simulink library "xbsDSP48_r3"  (Simulink 5.0)
libraries: xbsIndex_r3 x429, xbsDSP48_r3 x2
(part 2 of 8)

== system xbsDSP48_r3/DSP48_Adder ==
  note: A and C Type Casting : No Cost in Hardware
  note: Carry in Select Mux : From Fabric or no Carry in
  note: Output P Type Casting to  User Defined
      | Data Type
  In1 : Inport
  In3 : Inport  Port=2
  In6 : Inport  Port=3
  A : xbsIndex_r3/Slice  mode=Upper Bit Location + Width  nbits=18  bit1=0  base1=MSB of Input  bit0=0  base0=LSB of Input  boolean_output=off  explicit_period=off  period=1  dbl_ovrd=off
  AlignA : S-Function  AncestorBlock=xbsIndex_r3/Convert  FunctionName=xlconvert  Parameters=sfcn_mwsv__  mask(Xilinx Converter Block){arith_type=Signed  (2's comp), n_bits=15, bin_pt=0, quantization=Truncate, overflow=Wrap, latency=0, explicit_period=off, period=1, dbl_ovrd=off, show_param=off, inserted_by_tool=off, xl_area=[0, 0, 0, 0, 0, 0, 0], xl_use_area=off}
      mask prompts: arith_type "Output Type"; n_bits "Number of Bits"; bin_pt "Binary Point"; quantization "Quantization Behavior"; overflow "Overflow Behavior"; explicit_period "Use Explicit Sample Period"; period "Sample Period"; dbl_ovrd "Override with Doubles"; show_param "---------------------- Show Implementation Parameters -----------------------------------------------------------------------------------"; inserted_by_tool "Hidden Parameter:  inserted_by_tool"; xl_area "FPGA Area [Slices, FFs, BRAMs, LUTs, IOBs, Emb. Mults, TBUFs]"; xl_use_area "Use Area Above For Estimation"
      mask help:
      | Type conversion block. The input is presented at the output after quantization and overflow effects.
      |
      | Hardware notes: Additional hardware is used when rounding or saturation is selected and output width is less than the input width.
      mask init:
      | [designRoot, family, part, speed, package, simulinkPeriod, sysclkPeriod, dbl_ovrd, trimVbit] = xlSysgenSettings(gcb,1,1);
      | if (arith_type==1)
      |   bool = 1;
      | else
      |   bool = 0;
      |   arith_type = arith_type-1;
      | end
      | zstr=''; zpstr='';
      | if latency > 0
      |   zstr = 'z';
      |   zpstr = sprintf('-%d', latency);
      | end
      | [bg,fg] = xlcmap('XBlock',dbl_ovrd);
      | if (inserted_by_tool)
      |   bg = [1.00 0.50 0.25];
      | end
      | iPos = get_param(gcb,'Position');
      | iWidth=iPos(3)-iPos(1); iHeight=iPos(4)-iPos(2);
      | iCx=iWidth/2;
      | iCy=iHeight/2;
      | [logoX, logoY] = xlogo(iPos);
      | zstrx = 0.45*iWidth-11; if (zstrx<3) zstrx=3; end
      | zstry = 0.36*iHeight-7; if (zstry<3) zstry=3; end
      | 
      | 
      | % one time added for param list
      | dblOvrd = dbl_ovrd;
      | precision0 = 2;
      | z0 = [n_bits bin_pt arith_type quantization overflow];
      | explicitClk = explicit_period;
      | 
      | 
      | % just pass everything to s-function
      | sfcn_mwsv__ = get_param(gcb, 'MaskWSVariables');
      mask Help: web(xlhtmldoclink('Convert'));
      mask StyleString: popup(Boolean|Unsigned|Signed  (2's comp)),edit,edit,popup(Truncate|Round  (unbiased: +/- Inf)|Round  (unbiased: Even Values)),popup(Wrap|Saturate|Error),edit,checkbox,edit,checkbox,checkbox,checkbox,edit,checkbox
      mask Display:
      | patch([0 iWidth iWidth 0],[0 0 iHeight iHeight] , bg);
      | patch(logoX,logoY , fg);
      | text(zstrx,zstry,zstr);
      | text(zstrx+5,zstry+5,zpstr);
      | port_label('output',1,'cast');
      | plot([0 0 iWidth iWidth 0], [0 iHeight iHeight 0 0]);
  AlignC : xbsIndex_r3/Convert  arith_type="Signed  (2's comp)"  n_bits=12  bin_pt=0  quantization=Truncate  overflow=Wrap  latency=0  explicit_period=off  period=1  dbl_ovrd=off  show_param=off  inserted_by_tool=off  pipeline=off
      settings: xl_area=[0, 0, 0, 0, 0, 0, 0]
  AlignP : xbsIndex_r3/Reinterpret  force_arith_type=off  arith_type=Unsigned  force_bin_pt=on  bin_pt=0  force_valid=on
  B : xbsIndex_r3/Slice  mode=Lower Bit Location + Width  nbits=18  bit1=0  base1=MSB of Input  bit0=0  base0=LSB of Input  boolean_output=off  explicit_period=off  period=1  dbl_ovrd=off
  ConvertP : xbsIndex_r3/Convert  arith_type="Signed  (2's comp)"  n_bits=48  bin_pt=0  quantization=Truncate  overflow=Wrap  latency=0  explicit_period=off  period=1  dbl_ovrd=off  show_param=off  inserted_by_tool=off  pipeline=off
      settings: xl_area=[0, 0, 0, 0, 0, 0, 0]
  DSP48 : S-Function  FunctionName=xldsp48  Parameters=sfcn_mwsv__  mask(Xilinx DSP48){pipeline_a=1, use_b=Direct from B Port, pipeline_b=1, pipeline_bcin=0, pipeline_c=on, pipeline_p=on, pipeline_mult=on, pipeline_opmode=on, pipeline_sub=on, pipeline_carryin=on, pipeline_carryinsel=on, use_op=off, use_creg=on, use_pcin=off, use_pcout=off, use_bcout=off, access_rst=off, rst_all=off, rst_a=off, rst_b=off, rst_bcin=off, rst_c=off, rst_p=off, rst_mult=off, rst_carry_in=off, rst_ctrl=off, access_en=off, en_all=off, en_a=off, en_b=off, en_bcin=off, en_c=off, en_p=off, en_mult=off, en_carry_in=off, en_ctrl=off, explicit_period=off, period=1, dbl_ovrd=off, xl_area=[0, 0, 0, 0, 0, 0, 0], xl_use_area=on}
      mask prompts: pipeline_a "Pipeline Input A"; use_b "B Input"; pipeline_b "Pipeline Input B"; pipeline_bcin "Pipeline Input BCIN"; pipeline_c "Pipeline Input C"; pipeline_p "Pipeline P"; pipeline_mult "Pipeline Multiplier"; pipeline_opmode "Pipeline OpMode"; pipeline_sub "Pipeline Subtract"; pipeline_carryin "Pipeline Carry In"; pipeline_carryinsel "Pipeline Carry In Sel"; use_op "Consolidate Control Port (opmode, subtract, carry_in, carry_in_sel)"; use_creg "Provide C Port"; use_pcin "Provide PCIN Port"; use_pcout "Provide PCOUT Port"; use_bcout "Provide BCOUT Port"; access_rst "---------------------- Access Reset Port Control ---------------------------------------------------------"; rst_all "Provide Global Reset Port"; rst_a "Provide Reset Port for A"; rst_b "Provide Reset Port for B"; rst_bcin "Provide Reset Port for BCIN"; rst_c "Provide Reset Port for C"; rst_p "Provide Reset Port for P"; rst_mult "Provide Reset Port for Multiplier"; rst_carry_in "Provide Reset Port for Carry In"; rst_ctrl "Provide Reset Port for Controls (Subtract, CarryInSel, OpMode)"; access_en "---------------------- Access Enable Port Controls ---------------------------------------------------------"; en_all "Provide Global Enable Port"; en_a "Provide Enable Port for A"; en_b "Provide Enable Port for B"; en_bcin "Provide Enable Port for BCIN"; en_c "Provide Enable Port for C"; en_p "Provide Enable Port for P"; en_mult "Provide Enable Port for Multiplier"; en_carry_in "Provide Enable Port for Carry In"; en_ctrl "Provide Enable Port for Controls (Subtract, CarryInSel, OpMode)"; explicit_period "Use Explicit Sample Period"; period "Sample Period  (use -1 to inherit first known input period)"; dbl_ovrd "Override with Doubles"; xl_area "FPGA Area [Slices, FFs, BRAMs, LUTs, IOBs, Emb. Mults, TBUFs]"; xl_use_area "Use Area Above For Estimation"
      mask init:
      | [designRoot, family, part, speed, package, simulinkPeriod, sysclkPeriod, dbl_ovrd, trimVbit] = xlSysgenSettings(gcb,1,0);
      | trimVbit=1;
      | [bg,fg] = xlcmap('XBlock',dbl_ovrd);
      | iPos = get_param(gcb,'Position');
      | iWidth=iPos(3)-iPos(1); iHeight=iPos(4)-iPos(2);
      | iCx=iWidth/2;
      | iCy=iHeight/2;
      | [logoX, logoY] = xlogo(iPos);
      | opt_ports = 3; % default starting port num for optional ports
      | %initialize all the strings
      | b_str = 'a'; b_num = 1;
      | c_str = 'a'; c_num = 1;
      | ce_all_str = 'a'; rst_all_str = 'a';
      | ce_a_str = 'a'; rst_a_str = 'a';
      | ce_b_str = 'a'; rst_b_str = 'a';
      | ce_c_str = 'a'; rst_c_str = 'a';
      | ce_mult_str = 'a'; rst_mult_str = 'a';
      | ce_p_str = 'a'; rst_p_str = 'a';
      | ce_ctrl_str = 'a'; rst_ctrl_str = 'a';
      | ce_carryin_str = 'a'; rst_carryin_str = 'a';
      | ce_cinsub_str = 'a'; rst_cinsub_str = 'a';
      | bcin_str = 'a'; pcin_str = 'a';
      | pcout_str = 'p'; bcout_str = 'p';
      | opstr = 'a'; sub_str = 'a'; carryin_str = 'a';
      | carryin_sel_str = 'a';
      | % initialize all the port nums
      | ce_all_num = 1; rst_all_num = 1;
      | ce_a_num = 1; rst_a_num = 1;
      | ce_b_num = 1; rst_b_num = 1;
      | ce_c_num = 1; rst_c_num = 1;
      | ce_p_num = 1; rst_p_num = 1;
      | ce_mult_num = 1; rst_mult_num = 1;
      | ce_ctrl_num = 1; rst_ctrl_num = 1;
      | ce_carryin_num = 1; rst_carryin_num = 1;
      | ce_cinsub_num = 1; rst_cinsub_num = 1;
      | bcin_num = 1; pcin_num = 1;
      | pcout_num = 1; bcout_num = 1;
      | opnum = 1; sub_num = 1;
      | carryin_num = 1; carryin_sel_num = 1;
      | %Determine output ports
      | if(use_bcout == 1)
      | 	bcout_num = 2;
      | 	bcout_str = 'bcout';
      | end
      | if(use_pcout == 1)
      | 	if(use_bcout == 1)
      | 		pcout_num = 3;
      | 	else
      | 		pcout_num = 2;
      | 	end
      | 	pcout_str = 'pcout';
      | end
      | %determine to use b or bcin
      | if(use_b == 1) % USE B
      | 	b_str = 'b';
      | 	b_num = 2;
      | end
      | if(use_b == 2) % USE BCIN - place in same location as B
      | 	bcin_num = 2;
      | 	bcin_str = 'bcin';
      | end
      | if(use_creg == 1)
      | 	c_num = 3;
      | 	opt_ports = 4;
      | 	c_str = 'c';
      | end
      | if(use_pcin == 1)
      | 	pcin_num = opt_ports;
      | 	pcin_str = 'pcin';
      | 	opt_ports = opt_ports + 1;
      | end
      | %determine to use consolidated opmode or not
      | if(use_op == 1)
      | 	opnum = opt_ports;
      | 	opt_ports = opt_ports + 1;
      | 	opstr = 'op';
      | else
      | 	opnum = opt_ports;
      | 	opstr = 'opmode';
      | 	opt_ports = opt_ports + 1;
      | 	sub_num = opt_ports;
      | 	sub_str = 'subtract';
      | 	opt_ports = opt_ports + 1;
      | 	carryin_num = opt_ports;
      | 	carryin_str = 'carry_in';
      | 	opt_ports = opt_ports + 1;
      | 	carryin_sel_num = opt_ports;
      | 	carryin_sel_str = 'carry_in_sel';
      | 	opt_ports = opt_ports + 1;
      | end
      | %determine which optional ports to display
      | if(en_all == 1)
      | 	ce_a_str = 'en';
      | 	ce_a_num = opt_ports;
      | 	opt_ports = opt_ports + 1;
      | end
      | if(pipeline_a ~= 1 & en_a == 1 & en_all == 0)
      | 	ce_a_str = 'ce_a';
      | 	ce_a_num = opt_ports;
      | 	opt_ports = opt_ports + 1;
      | end
      | if(pipeline_b ~= 1 & (en_b == 1 || en_bcin == 1) & en_all == 0)
      | 	if(en_b == 1)
      | 		ce_b_str = 'ce_b';
      | 	end
      | 	if(en_bcin == 1)
      | 		ce_b_str = 'ce_bcin';
      | 	end
      | 	ce_b_num = opt_ports;
      | 	opt_ports = opt_ports + 1;
      | end
      | if(pipeline_c == 1 & en_c == 1 & en_all == 0)
      | 	ce_c_num = opt_ports;
      | 	ce_c_str = 'ce_c';
      | 	opt_ports = opt_ports + 1;
      | end
      | if(pipeline_mult == 1 & en_mult == 1 & en_all == 0)
      | 	ce_mult_num = opt_ports;
      | 	ce_mult_str = 'ce_m';
      | 	opt_ports = opt_ports + 1;
      | end
      | if(pipeline_p == 1 & en_p == 1 & en_all == 0)
      | 	ce_p_num = opt_ports;
      | 	ce_p_str = 'ce_p';
      | 	opt_ports = opt_ports + 1;
      | end	
      | if(en_ctrl == 1 & en_all == 0)
      | 	ce_ctrl_str = 'ce_ctrl';
      | 	ce_ctrl_num = opt_ports;
      | 	opt_ports = opt_ports + 1;
      | end
      | if(en_carry_in == 1 & en_all == 0)
      | 	ce_carryin_num = opt_ports;
      | 	ce_carryin_str = 'ce_carry_in';
      | 	opt_ports = opt_ports + 1;
      | end
      | if(en_ctrl == 1 & en_all == 0)
      | 	ce_cinsub_str = 'ce_cinsub';
      | 	ce_cinsub_num = opt_ports;
      | 	opt_ports = opt_ports + 1;
      | end
      | %determine which rst ports to display
      | if(rst_all == 1)
      | 	rst_a_str = 'rst';
      | 	rst_a_num = opt_ports;
      | 	opt_ports = opt_ports + 1;
      | end
      | if(pipeline_a ~= 1 & rst_a == 1 & rst_all == 0)
      | 	rst_a_str = 'rst_a';
      | 	rst_a_num = opt_ports;
      | 	opt_ports = opt_ports + 1;
      | end
      | if(pipeline_b ~= 1 & (rst_b == 1|| rst_bcin) & rst_all == 0)
      | 	if(rst_b == 1)
      | 		rst_b_str = 'rst_b';
      | 	end
      | 	if(rst_bcin == 1)
      | 		rst_b_str = 'rst_bcin';
      | 	end
      | 	rst_b_num = opt_ports;
      | 	opt_ports = opt_ports + 1;
      | end
      | if(pipeline_c == 1 & rst_c == 1 & rst_all == 0)
      | 	rst_c_num = opt_ports;
      | 	rst_c_str = 'rst_c';
      | 	opt_ports = opt_ports + 1;
      | end
      | if(pipeline_mult == 1 & rst_mult == 1 & rst_all == 0)
      | 	rst_mult_num = opt_ports;
      | 	rst_mult_str = 'rst_m';
      | 	opt_ports = opt_ports + 1;
      | end
      | if(pipeline_p == 1 & rst_p == 1 & rst_all == 0)
      | 	rst_p_num = opt_ports;
      | 	rst_p_str = 'rst_p';
      | 	opt_ports = opt_ports + 1;
      | end
      | if(rst_ctrl == 1 & rst_all == 0)
      | 	rst_ctrl_str = 'rst_ctrl';
      | 	rst_ctrl_num = opt_ports;
      | 	opt_ports = opt_ports + 1;
      | end
      | if(rst_carry_in == 1 & rst_all == 0) 
      | rst_carryin_num = opt_ports;
      | rst_carryin_str = 'rst_carry_in';
      | opt_ports = opt_ports + 1;
      | end
      | 
      | % one time added for param list
      | latency = 1;
      | dblOvrd = dbl_ovrd;
      | precision0 = 1;
      | precision1 = 1;
      | precision2 = 1;
      | precision3 = 1;
      | precision4 = 1;
      | precision5 = 1;
      | precision6 = 1;
      | precision7 = 1;
      | precision8 = 1;
      | precision9 = 1;
      | precision10 = 1;
      | precision11 = 1;
      | precision12 = 1;
      | precision13 = 1;
      | precision14 = 1;
      | precision15 = 1;
      | precision16 = 1;
      | precision17 = 1;
      | precision18 = 1;
      | precision19 = 1;
      | precision20 = 1;
      | precision21 = 1;
      | precision22 = 1;
      | precision23 = 1;
      | precision24 = 1;
      | precision25 = 1;
      | precision26 = 1;
      | explicitClk = explicit_period;
      | hasEN = 0;
      | hasRST = 0;
      | % just pass everything to s-function
      | sfcn_mwsv__ = get_param(gcb, 'MaskWSVariables');
      mask Help: web(xlhtmldoclink('DSP48'));
      mask StyleString: popup(0|1|2),popup(Direct from B Port|Cascaded from BCIN Port),popup(0|1|2),popup(0|1|2),checkbox,checkbox,checkbox,checkbox,checkbox,checkbox,checkbox,checkbox,checkbox,checkbox,checkbox,checkbox,checkbox,checkbox,checkbox,checkbox,checkbox,checkbox,checkbox,checkbox,checkbox,checkbox,checkbox,checkbox,checkbox,checkbox,checkbox,checkbox,checkbox,checkbox,checkbox,checkbox,checkbox,edit,checkbox,edit,checkbox
      mask Display:
      | patch([0 iWidth iWidth 0],[0 0 iHeight iHeight] , bg);
      | patch(logoX,logoY , fg);
      | port_label('input',1,'a');
      | port_label('input',b_num,b_str);
      | port_label('input',c_num,c_str);
      | port_label('input',opnum,opstr);
      | port_label('input',sub_num,sub_str);
      | port_label('input',carryin_num,carryin_str);
      | port_label('input',carryin_sel_num,carryin_sel_str);
      | port_label('input',ce_a_num,ce_a_str);
      | port_label('input',ce_b_num,ce_b_str);
      | port_label('input',ce_c_num,ce_c_str);
      | port_label('input',ce_mult_num,ce_mult_str);
      | port_label('input',ce_p_num,ce_p_str);
      | port_label('input',ce_ctrl_num,ce_ctrl_str);
      | port_label('input',ce_carryin_num,ce_carryin_str);
      | port_label('input',ce_cinsub_num,ce_cinsub_str);
      | port_label('input',rst_a_num,rst_a_str);
      | port_label('input',rst_b_num,rst_b_str);
      | port_label('input',rst_c_num,rst_c_str);
      | port_label('input',rst_mult_num,rst_mult_str);
      | port_label('input',rst_p_num,rst_p_str);
      | port_label('input',rst_ctrl_num,rst_ctrl_str);
      | port_label('input',rst_carryin_num,rst_carryin_str);
      | port_label('input',bcin_num,bcin_str);
      | port_label('input',pcin_num,pcin_str);
      | port_label('output',bcout_num,bcout_str );
      | port_label('output',pcout_num,pcout_str);
      | port_label('output',1,'p');
      | plot([0 0 iWidth iWidth 0], [0 iHeight iHeight 0 0]);
  Mux : xbsIndex_r3/Mux  inputs=2  precision=Full  arith_type="Signed  (2's comp)"  n_bits=8  bin_pt=2  quantization=Truncate  overflow=Wrap  latency=0  explicit_period=off  period=1  en=off  dbl_ovrd=off  show_param=off  mux_type=off  use_rpm=off  gen_core=off
      settings: xl_area=[0, 0, 0, 0, 0, 0, 0]
  PrecA : xbsIndex_r3/Convert  arith_type="Signed  (2's comp)"  n_bits=36  bin_pt=0  quantization=Truncate  overflow=Wrap  latency=0  explicit_period=off  period=1  dbl_ovrd=off  show_param=off  inserted_by_tool=off  pipeline=off
      settings: xl_area=[0, 0, 0, 0, 0, 0, 0]
  PrecA2 : xbsIndex_r3/Convert  arith_type="Signed  (2's comp)"  n_bits=18  bin_pt=0  quantization=Truncate  overflow=Wrap  latency=0  explicit_period=off  period=1  dbl_ovrd=off  show_param=off  inserted_by_tool=off  pipeline=off
      settings: xl_area=[0, 0, 0, 0, 0, 0, 0]
  PrecB2 : xbsIndex_r3/Convert  arith_type="Signed  (2's comp)"  n_bits=18  bin_pt=0  quantization=Truncate  overflow=Wrap  latency=0  explicit_period=off  period=1  dbl_ovrd=off  show_param=off  inserted_by_tool=off  pipeline=off
      settings: xl_area=[0, 0, 0, 0, 0, 0, 0]
  PrecC : xbsIndex_r3/Convert  arith_type="Signed  (2's comp)"  n_bits=48  bin_pt=0  quantization=Truncate  overflow=Wrap  latency=0  explicit_period=off  period=1  dbl_ovrd=off  show_param=off  inserted_by_tool=off  pipeline=off
      settings: xl_area=[0, 0, 0, 0, 0, 0, 0]
  ReinterpretA : xbsIndex_r3/Reinterpret  force_arith_type=off  arith_type=Unsigned  force_bin_pt=on  bin_pt=0  force_valid=on
  ReinterpretC : xbsIndex_r3/Reinterpret  force_arith_type=off  arith_type=Unsigned  force_bin_pt=on  bin_pt=0  force_valid=on
  UDType : xbsIndex_r3/Convert  arith_type="Signed  (2's comp)"  n_bits=48  bin_pt=0  quantization=Truncate  overflow=Wrap  latency=0  explicit_period=off  period=1  dbl_ovrd=off  show_param=off  inserted_by_tool=off  pipeline=off
      settings: xl_area=[0, 0, 0, 0, 0, 0, 0]
  carry_in_sel : xbsIndex_r3/Constant  const=0  arith_type=Unsigned  n_bits=2  bin_pt=0  explicit_period=off  period=1  dbl_ovrd=off
  carry_sel : xbsIndex_r3/Constant  const=1  equ=P=C  arith_type=Unsigned  n_bits=1  bin_pt=0  opselect=C  inp2=PCIN>>17  opr=+  inp1=P  carry=CIN  iostate=0  explicit_period=off  period=1  dbl_ovrd=off
  no_carry : xbsIndex_r3/Constant  const=0  arith_type=Boolean  n_bits=2  bin_pt=0  explicit_period=off  period=1  dbl_ovrd=off
  opmode : Subsystem
  subtract : xbsIndex_r3/Constant  const=0  equ=P=C  arith_type=Boolean  n_bits=1  bin_pt=0  opselect=C  inp2=PCIN>>17  opr=+  inp1=P  carry=CIN  iostate=0  explicit_period=off  period=1  dbl_ovrd=off
  Out1 : Outport
  wires:
  In1/1 -> AlignA/1
  In3/1 -> AlignC/1
  opmode/1(op) -> DSP48/4
  DSP48/1 -> ConvertP/1
  AlignA/1 -> ReinterpretA/1
  B/1 -> PrecB2/1
  A/1 -> PrecA2/1
  AlignC/1 -> ReinterpretC/1
  subtract/1 -> DSP48/5
  carry_in_sel/1 -> DSP48/7
  ConvertP/1 -> AlignP/1
  PrecA/1 -> B/1, A/1
  ReinterpretA/1 -> PrecA/1
  ReinterpretC/1 -> PrecC/1
  PrecC/1 -> DSP48/3
  PrecA2/1 -> DSP48/1
  PrecB2/1 -> DSP48/2
  AlignP/1 -> UDType/1
  UDType/1 -> Out1/1
  In6/1 -> Mux/3
  Mux/1 -> DSP48/6
  no_carry/1 -> Mux/2
  carry_sel/1 -> Mux/1

== system xbsDSP48_r3/DSP48_Mult ==
  note: Casting A and B for Using DSP 48 BlockA and B Donot need to
      | be aligned befor Multiplication
  note: C is aligned with respect to A*B data presented to the Adder
      |  within DSP48
  note: Carry in Select Mux : From Fabric or no Carry in
  note: Aligning and Casting to a User defined data type
  In1 : Inport
  In2 : Inport  Port=2
  In3 : Inport  Port=3
  In6 : Inport  Port=4
  AlignA : xbsIndex_r3/Convert  arith_type="Signed  (2's comp)"  n_bits=10  bin_pt=0  quantization=Truncate  overflow=Wrap  latency=0  explicit_period=off  period=1  dbl_ovrd=off  show_param=off  inserted_by_tool=off  pipeline=off
      settings: xl_area=[0, 0, 0, 0, 0, 0, 0]
  AlignB : xbsIndex_r3/Convert  arith_type="Signed  (2's comp)"  n_bits=14  bin_pt=0  quantization=Truncate  overflow=Wrap  latency=0  explicit_period=off  period=1  dbl_ovrd=off  show_param=off  inserted_by_tool=off  pipeline=off
      settings: xl_area=[0, 0, 0, 0, 0, 0, 0]
  AlignC : xbsIndex_r3/Convert  arith_type="Signed  (2's comp)"  n_bits=24  bin_pt=0  quantization=Truncate  overflow=Wrap  latency=0  explicit_period=off  period=1  dbl_ovrd=off  show_param=off  inserted_by_tool=off  pipeline=off
      settings: xl_area=[0, 0, 0, 0, 0, 0, 0]
  CastP : xbsIndex_r3/Convert  arith_type="Signed  (2's comp)"  n_bits=48  bin_pt=0  quantization=Truncate  overflow=Wrap  latency=0  explicit_period=off  period=1  dbl_ovrd=off  show_param=off  inserted_by_tool=off
      settings: xl_area=[0, 0, 0, 0, 0, 0, 0]
  DSP48 : xbsIndex_r3/DSP48  pipeline_a=1  use_b=Direct from B Port  pipeline_b=1  pipeline_bcin=2  pipeline_c=on  pipeline_p=on  pipeline_mult=on  pipeline_opmode=on  pipeline_sub=on  pipeline_carryin=on  pipeline_carryinsel=on  use_op=off  use_creg=on  use_pcin=off  use_pcout=off  use_bcout=off  access_rst=off  rst_all=off  rst_a=off  rst_b=off  rst_bcin=off  rst_c=off  rst_p=off  rst_mult=off  rst_carry_in=off  rst_ctrl=off  access_en=off  en_all=off  en_a=off  en_b=off  en_bcin=off  en_c=off  en_p=off  en_mult=off  en_carry_in=off  en_ctrl=off  explicit_period=off  period=1  dbl_ovrd=off
      settings: xl_area=[0, 0, 0, 0, 0, 0, 0]  xl_use_area=on
  FullP : xbsIndex_r3/Reinterpret  force_arith_type=on  arith_type=Unsigned  force_bin_pt=on  bin_pt=0  force_valid=on
  Mux : xbsIndex_r3/Mux  inputs=2  precision=Full  arith_type="Signed  (2's comp)"  n_bits=8  bin_pt=2  quantization=Truncate  overflow=Wrap  latency=0  explicit_period=off  period=1  en=off  dbl_ovrd=off  show_param=off  mux_type=off  use_rpm=off  gen_core=off
      settings: xl_area=[0, 0, 0, 0, 0, 0, 0]
  PrecA : xbsIndex_r3/Convert  arith_type="Signed  (2's comp)"  n_bits=18  bin_pt=0  quantization=Truncate  overflow=Wrap  latency=0  explicit_period=off  period=1  dbl_ovrd=off  show_param=off  inserted_by_tool=off
      settings: xl_area=[0, 0, 0, 0, 0, 0, 0]
  PrecB : xbsIndex_r3/Convert  arith_type="Signed  (2's comp)"  n_bits=18  bin_pt=0  quantization=Truncate  overflow=Wrap  latency=0  explicit_period=off  period=1  dbl_ovrd=off  show_param=off  inserted_by_tool=off
      settings: xl_area=[0, 0, 0, 0, 0, 0, 0]
  PrecC : xbsIndex_r3/Convert  arith_type="Signed  (2's comp)"  n_bits=48  bin_pt=0  quantization=Truncate  overflow=Wrap  latency=0  explicit_period=off  period=1  dbl_ovrd=off  show_param=off  inserted_by_tool=off
      settings: xl_area=[0, 0, 0, 0, 0, 0, 0]
  ReinterpretA : xbsIndex_r3/Reinterpret  force_arith_type=off  arith_type=Unsigned  force_bin_pt=on  bin_pt=0  force_valid=on
  ReinterpretB : xbsIndex_r3/Reinterpret  force_arith_type=off  arith_type=Unsigned  force_bin_pt=on  bin_pt=0  force_valid=on
  ReinterpretC : xbsIndex_r3/Reinterpret  force_arith_type=off  arith_type=Unsigned  force_bin_pt=on  bin_pt=0  force_valid=on
  UDTypeP : xbsIndex_r3/Convert  arith_type="Signed  (2's comp)"  n_bits=48  bin_pt=0  quantization=Truncate  overflow=Wrap  latency=0  explicit_period=off  period=1  dbl_ovrd=off  show_param=off  inserted_by_tool=off  pipeline=off
      settings: xl_area=[0, 0, 0, 0, 0, 0, 0]
  carry_in_sel : xbsIndex_r3/Constant  const=0  arith_type=Unsigned  n_bits=2  bin_pt=0  explicit_period=off  period=1  dbl_ovrd=off
  carry_sel : xbsIndex_r3/Constant  const=1  equ=P=C  arith_type=Unsigned  n_bits=1  bin_pt=0  opselect=C  inp2=PCIN>>17  opr=+  inp1=P  carry=CIN  iostate=0  explicit_period=off  period=1  dbl_ovrd=off
  no_carry : xbsIndex_r3/Constant  const=0  arith_type=Boolean  n_bits=2  bin_pt=0  explicit_period=off  period=1  dbl_ovrd=off
  opmode : Subsystem
  subtract : xbsIndex_r3/Constant  const=0  equ=P=C  arith_type=Boolean  n_bits=1  bin_pt=0  opselect=C  inp2=PCIN>>17  opr=+  inp1=P  carry=CIN  iostate=0  explicit_period=off  period=1  dbl_ovrd=off
  Out1 : Outport
  wires:
  In1/1 -> AlignA/1
  In3/1 -> AlignC/1
  opmode/1(op) -> DSP48/4
  DSP48/1 -> CastP/1
  carry_in_sel/1 -> DSP48/7
  CastP/1 -> FullP/1
  In2/1 -> AlignB/1
  ReinterpretA/1 -> PrecA/1
  PrecA/1 -> DSP48/1
  ReinterpretB/1 -> PrecB/1
  PrecB/1 -> DSP48/2
  AlignC/1 -> ReinterpretC/1
  ReinterpretC/1 -> PrecC/1
  AlignA/1 -> ReinterpretA/1
  AlignB/1 -> ReinterpretB/1
  no_carry/1 -> Mux/2
  carry_sel/1 -> Mux/1
  subtract/1 -> DSP48/5
  Mux/1 -> DSP48/6
  In6/1 -> Mux/3
  FullP/1 -> UDTypeP/1
  UDTypeP/1 -> Out1/1
  PrecC/1 -> DSP48/3

== system xbsDSP48_r3/DSP48reg ==
  d : Inport
  rst : Inport  Port=2
  ce : Inport  Port=3
  Register1 : xbsIndex_r3/Register  init=0  reg_only_valid=off  explicit_period=off  period=1  rst=on  en=on  out_en=off  dbl_ovrd=off  show_param=off
      settings: xl_area=[0, 0, 0, 0, 0, 0, 0]
  q : Outport
  wires:
  d/1 -> Register1/1
  rst/1 -> Register1/2
  ce/1 -> Register1/3
  Register1/1 -> q/1

== system xbsDSP48_r3/MultTemplate ==
  In1 : Inport
  In2 : Inport  Port=2
  In3 : Inport  Port=3
  In4 : Inport  Port=4
  In5 : Inport  Port=5
  In6 : Inport  Port=6
  In7 : Inport  Port=7
  AlignP : xbsIndex_r3/Reinterpret  force_arith_type=on  arith_type=Unsigned  force_bin_pt=on  bin_pt=0  force_valid=on
  ConvertP : xbsIndex_r3/Convert  arith_type="Signed  (2's comp)"  n_bits=48  bin_pt=0  quantization=Truncate  overflow=Wrap  latency=0  explicit_period=off  period=1  dbl_ovrd=off  show_param=off  inserted_by_tool=off  pipeline=off
      settings: xl_area=[0, 0, 0, 0, 0, 0, 0]
  DSP48 : xbsIndex_r3/DSP48  pipeline_a=1  use_b=Direct from B Port  pipeline_b=1  pipeline_bcin=0  pipeline_c=on  pipeline_p=on  pipeline_mult=on  pipeline_opmode=on  pipeline_sub=on  pipeline_carryin=on  pipeline_carryinsel=on  use_op=off  use_creg=on  use_pcin=off  use_pcout=off  use_bcout=off  access_rst=off  rst_all=off  rst_a=off  rst_b=off  rst_bcin=off  rst_c=off  rst_p=off  rst_mult=off  rst_carry_in=off  rst_ctrl=off  access_en=off  en_all=off  en_a=off  en_b=off  en_bcin=off  en_c=off  en_p=off  en_mult=off  en_carry_in=off  en_ctrl=off  explicit_period=off  period=1  dbl_ovrd=off
      settings: xl_area=[0, 0, 0, 0, 0, 0, 0]  xl_use_area=on
  UDType : xbsIndex_r3/Convert  arith_type="Signed  (2's comp)"  n_bits=48  bin_pt=0  quantization=Truncate  overflow=Wrap  latency=0  explicit_period=off  period=1  dbl_ovrd=off  show_param=off  inserted_by_tool=off  pipeline=off
      settings: xl_area=[0, 0, 0, 0, 0, 0, 0]
  Out1 : Outport
  wires:
  DSP48/1 -> ConvertP/1
  ConvertP/1 -> AlignP/1
  AlignP/1 -> UDType/1
  UDType/1 -> Out1/1
  In3/1 -> DSP48/4
  In4/1 -> DSP48/5
  In6/1 -> DSP48/7
  In5/1 -> DSP48/6
  In2/1 -> DSP48/3
  In1/1 -> DSP48/1
  In7/1 -> DSP48/2

== system xbsDSP48_r3/MultTemplatenc ==
  In1 : Inport
  In2 : Inport  Port=2
  In3 : Inport  Port=3
  In4 : Inport  Port=4
  In5 : Inport  Port=5
  In6 : Inport  Port=6
  In7 : Inport  Port=7
  AlignP : xbsIndex_r3/Reinterpret  force_arith_type=on  arith_type=Unsigned  force_bin_pt=on  bin_pt=0  force_valid=on
  ConvertP : xbsIndex_r3/Convert  arith_type="Signed  (2's comp)"  n_bits=48  bin_pt=0  quantization=Truncate  overflow=Wrap  latency=0  explicit_period=off  period=1  dbl_ovrd=off  show_param=off  inserted_by_tool=off  pipeline=off
      settings: xl_area=[0, 0, 0, 0, 0, 0, 0]
  DSP48 : xbsIndex_r3/DSP48  pipeline_a=1  use_b=Direct from B Port  pipeline_b=1  pipeline_bcin=0  pipeline_c=on  pipeline_p=on  pipeline_mult=on  pipeline_opmode=on  pipeline_sub=on  pipeline_carryin=on  pipeline_carryinsel=on  use_op=off  use_creg=off  use_pcin=off  use_pcout=off  use_bcout=off  access_rst=off  rst_all=off  rst_a=off  rst_b=off  rst_bcin=off  rst_c=off  rst_mult=off  rst_p=off  rst_ctrl=off  rst_carry_in=off  access_en=off  en_all=off  en_a=off  en_b=off  en_bcin=off  en_c=off  en_mult=off  en_p=off  en_carry_in=off  en_ctrl=off  explicit_period=off  period=1  dbl_ovrd=off
      settings: xl_area=[0, 0, 0, 0, 0, 0, 0]  xl_use_area=on
  Terminator : Terminator
  UDType : xbsIndex_r3/Convert  arith_type="Signed  (2's comp)"  n_bits=48  bin_pt=0  quantization=Truncate  overflow=Wrap  latency=0  explicit_period=off  period=1  dbl_ovrd=off  show_param=off  inserted_by_tool=off  pipeline=off
      settings: xl_area=[0, 0, 0, 0, 0, 0, 0]
  Out1 : Outport
  wires:
  DSP48/1 -> ConvertP/1
  ConvertP/1 -> AlignP/1
  AlignP/1 -> UDType/1
  UDType/1 -> Out1/1
  In1/1 -> DSP48/1
  In7/1 -> DSP48/2
  In3/1 -> DSP48/3
  In4/1 -> DSP48/4
  In5/1 -> DSP48/5
  In6/1 -> DSP48/6
  In2/1 -> Terminator/1

== system xbsDSP48_r3/vAdderTemplate ==
  In1 : Inport
  In2 : Inport  Port=2
  In3 : Inport  Port=3
  In4 : Inport  Port=4
  In5 : Inport  Port=5
  In6 : Inport  Port=6
  ASlice : xbsIndex_r3/Slice  mode=Upper Bit Location + Width  nbits=18  bit1=0  base1=MSB of Input  bit0=0  base0=LSB of Input  boolean_output=off  explicit_period=off  period=1  dbl_ovrd=off
  AlignP : xbsIndex_r3/Reinterpret  force_arith_type=off  arith_type=Unsigned  force_bin_pt=on  bin_pt=0  force_valid=on
  BSlice : xbsIndex_r3/Slice  mode=Lower Bit Location + Width  nbits=18  bit1=0  base1=MSB of Input  bit0=0  base0=LSB of Input  boolean_output=off  explicit_period=off  period=1  dbl_ovrd=off
  ConvertP : xbsIndex_r3/Convert  arith_type="Signed  (2's comp)"  n_bits=48  bin_pt=0  quantization=Truncate  overflow=Wrap  latency=0  explicit_period=off  period=1  dbl_ovrd=off  show_param=off  inserted_by_tool=off  pipeline=off
      settings: xl_area=[0, 0, 0, 0, 0, 0, 0]
  DSP48 : Subsystem  mask(Xilinx vDSP48){pipeline_a=1, use_b=Direct from B port, pipeline_b=1, pipeline_bcin=0, pipeline_c=on, pipeline_p=on, pipeline_mult=on, pipeline_opmode=on, pipeline_sub=on, pipeline_carryin=on, pipeline_carryinsel=on, use_creg=on, use_pcin=off, use_pcout=off, use_bcout=off, access_rst=on, rst_all=off, rst_a=off, rst_b=off, rst_c=off, rst_p=off, rst_mult=off, rst_carry_in=off, rst_ctrl=off, access_en=on, en_all=off, en_a=off, en_b=off, en_c=off, en_p=off, en_mult=off, en_carry_in=off, en_ctrl=off, period=2, statestr=|1|Direct from B port|1|0|on|on|on|on|on|on|on|on|off|off|off|on|off|off|off|off|off|off|off|off|on|off|off|off|off|off|off|off|off|2}
      mask prompts: pipeline_a "Pipeline Input A"; use_b "B Input"; pipeline_b "Pipeline Input B"; pipeline_bcin "Pipeline Input BCIN"; pipeline_c "Pipeline Input C"; pipeline_p "Pipeline P"; pipeline_mult "Pipeline Multiplier"; pipeline_opmode "Pipeline Opmode"; pipeline_sub "Pipeline Subtract"; pipeline_carryin "Pipeline Carry In"; pipeline_carryinsel "Pipeline Carry In Sel"; use_creg "Provide C port"; use_pcin "Provide PCIN port"; use_pcout "Provide PCOUT port"; use_bcout "Provide BCOUT"; access_rst "---------------------------Access Reset Port Control------------------------------------"; rst_all "Provide Global Reset Port"; rst_a "Provide Reset Port for A"; rst_b "Provide Reset Port for B"; rst_c "Provide Reset Port for C"; rst_p "Provide Reset Port for P"; rst_mult "Provide Reset Port for Multiplier"; rst_carry_in "Provide Reset Port for Carry In"; rst_ctrl "Provide Reset Port for Controls (Subtract, CarryInSel, OpMode)"; access_en "----------------------------Access Enable Port Control---------------------------------"; en_all "Provide Global Enable Port"; en_a "Provide Enable for Port A"; en_b "Provide Enable for Port B"; en_c "Provide Enable for Port C"; en_p "Provide Enable for Port P"; en_mult "Provide Enable for Multiplier"; en_carry_in "Provide Enable for Carry In"; en_ctrl "Provide Enable Port for Controls (Subtract, CarryInSel, OpMode)"; period "Sample Period"
      mask init:
      | this_gcb = gcb;
      | set_param(this_gcb,'linkstatus','none');
      | xlgenvDSP48callback(this_gcb);
      mask StyleString: popup(0|1|2),popup(Direct from B port|Cascaded from BCIN port),popup(0|1|2),popup(0|1|2),checkbox,checkbox,checkbox,checkbox,checkbox,checkbox,checkbox,checkbox,checkbox,checkbox,checkbox,checkbox,checkbox,checkbox,checkbox,checkbox,checkbox,checkbox,checkbox,checkbox,checkbox,checkbox,checkbox,checkbox,checkbox,checkbox,checkbox,checkbox,checkbox,edit,edit
  PrecA1 : xbsIndex_r3/Convert  arith_type="Signed  (2's comp)"  n_bits=18  bin_pt=0  quantization=Truncate  overflow=Wrap  latency=0  explicit_period=off  period=1  dbl_ovrd=off  show_param=off  inserted_by_tool=off  pipeline=off
      settings: xl_area=[0, 0, 0, 0, 0, 0, 0]
  PrecB1 : xbsIndex_r3/Convert  arith_type="Signed  (2's comp)"  n_bits=18  bin_pt=0  quantization=Truncate  overflow=Wrap  latency=0  explicit_period=off  period=1  dbl_ovrd=off  show_param=off  inserted_by_tool=off  pipeline=off
      settings: xl_area=[0, 0, 0, 0, 0, 0, 0]
  UDType : xbsIndex_r3/Convert  arith_type="Signed  (2's comp)"  n_bits=48  bin_pt=0  quantization=Truncate  overflow=Wrap  latency=0  explicit_period=off  period=1  dbl_ovrd=off  show_param=off  inserted_by_tool=off  pipeline=off
      settings: xl_area=[0, 0, 0, 0, 0, 0, 0]
  Out1 : Outport
  wires:
  In1/1 -> ASlice/1, BSlice/1
  PrecB1/1 -> DSP48/2(b)
  PrecA1/1 -> DSP48/1(a)
  ASlice/1 -> PrecA1/1
  BSlice/1 -> PrecB1/1
  AlignP/1 -> UDType/1
  UDType/1 -> Out1/1
  ConvertP/1 -> AlignP/1
  In2/1 -> DSP48/3(c)
  In3/1 -> DSP48/4(opmode)
  In4/1 -> DSP48/5(subtract)
  In5/1 -> DSP48/6(carry_in)
  In6/1 -> DSP48/7(carry_in_sel)
  DSP48/1(P) -> ConvertP/1

== system xbsDSP48_r3/vAdderTemplatenc ==
  In1 : Inport
  In2 : Inport  Port=2
  In3 : Inport  Port=3
  In4 : Inport  Port=4
  In5 : Inport  Port=5
  In6 : Inport  Port=6
  ASlice : xbsIndex_r3/Slice  mode=Upper Bit Location + Width  nbits=18  bit1=0  base1=MSB of Input  bit0=0  base0=LSB of Input  boolean_output=off  explicit_period=off  period=1  dbl_ovrd=off
  AlignP : xbsIndex_r3/Reinterpret  force_arith_type=off  arith_type=Unsigned  force_bin_pt=on  bin_pt=0  force_valid=on
  BSlice : xbsIndex_r3/Slice  mode=Lower Bit Location + Width  nbits=18  bit1=0  base1=MSB of Input  bit0=0  base0=LSB of Input  boolean_output=off  explicit_period=off  period=1  dbl_ovrd=off
  ConvertP : xbsIndex_r3/Convert  arith_type="Signed  (2's comp)"  n_bits=48  bin_pt=0  quantization=Truncate  overflow=Wrap  latency=0  explicit_period=off  period=1  dbl_ovrd=off  show_param=off  inserted_by_tool=off  pipeline=off
      settings: xl_area=[0, 0, 0, 0, 0, 0, 0]
  DSP48 : Subsystem  mask(Xilinx vDSP48){pipeline_a=1, use_b=Direct from B port, pipeline_b=1, pipeline_bcin=0, pipeline_c=on, pipeline_p=on, pipeline_mult=on, pipeline_opmode=on, pipeline_sub=on, pipeline_carryin=on, pipeline_carryinsel=on, use_creg=off, use_pcin=off, use_pcout=off, use_bcout=off, access_rst=on, rst_all=off, rst_a=off, rst_b=off, rst_c=off, rst_p=off, rst_mult=off, rst_carry_in=off, rst_ctrl=off, access_en=on, en_all=off, en_a=off, en_b=off, en_c=off, en_p=off, en_mult=off, en_carry_in=off, en_ctrl=off, period=1, statestr=|1|Direct from B port|1|0|on|on|on|on|on|on|on|off|off|off|off|on|off|off|off|off|off|off|off|off|on|off|off|off|off|off|off|off|off|1}
      mask prompts: pipeline_a "Pipeline Input A"; use_b "B Input"; pipeline_b "Pipeline Input B"; pipeline_bcin "Pipeline Input BCIN"; pipeline_c "Pipeline Input C"; pipeline_p "Pipeline P"; pipeline_mult "Pipeline Multiplier"; pipeline_opmode "Pipeline Opmode"; pipeline_sub "Pipeline Subtract"; pipeline_carryin "Pipeline Carry In"; pipeline_carryinsel "Pipeline Carry In Sel"; use_creg "Provide C port"; use_pcin "Provide PCIN port"; use_pcout "Provide PCOUT port"; use_bcout "Provide BCOUT"; access_rst "---------------------------Access Reset Port Control------------------------------------"; rst_all "Provide Global Reset Port"; rst_a "Provide Reset Port for A"; rst_b "Provide Reset Port for B"; rst_c "Provide Reset Port for C"; rst_p "Provide Reset Port for P"; rst_mult "Provide Reset Port for Multiplier"; rst_carry_in "Provide Reset Port for Carry In"; rst_ctrl "Provide Reset Port for Controls (Subtract, CarryInSel, OpMode)"; access_en "----------------------------Access Enable Port Control---------------------------------"; en_all "Provide Global Enable Port"; en_a "Provide Enable for Port A"; en_b "Provide Enable for Port B"; en_c "Provide Enable for Port C"; en_p "Provide Enable for Port P"; en_mult "Provide Enable for Multiplier"; en_carry_in "Provide Enable for Carry In"; en_ctrl "Provide Enable Port for Controls (Subtract, CarryInSel, OpMode)"; period "Sample Period"
      mask init:
      | this_gcb = gcb;
      | set_param(this_gcb,'linkstatus','none');
      | xlgenvDSP48callback(this_gcb);
      mask StyleString: popup(0|1|2),popup(Direct from B port|Cascaded from BCIN port),popup(0|1|2),popup(0|1|2),checkbox,checkbox,checkbox,checkbox,checkbox,checkbox,checkbox,checkbox,checkbox,checkbox,checkbox,checkbox,checkbox,checkbox,checkbox,checkbox,checkbox,checkbox,checkbox,checkbox,checkbox,checkbox,checkbox,checkbox,checkbox,checkbox,checkbox,checkbox,checkbox,edit,edit
  PrecA1 : xbsIndex_r3/Convert  arith_type="Signed  (2's comp)"  n_bits=18  bin_pt=0  quantization=Truncate  overflow=Wrap  latency=0  explicit_period=off  period=1  dbl_ovrd=off  show_param=off  inserted_by_tool=off  pipeline=off
      settings: xl_area=[0, 0, 0, 0, 0, 0, 0]
  PrecB1 : xbsIndex_r3/Convert  arith_type="Signed  (2's comp)"  n_bits=18  bin_pt=0  quantization=Truncate  overflow=Wrap  latency=0  explicit_period=off  period=1  dbl_ovrd=off  show_param=off  inserted_by_tool=off  pipeline=off
      settings: xl_area=[0, 0, 0, 0, 0, 0, 0]
  Terminator : Terminator
  UDType : xbsIndex_r3/Convert  arith_type="Signed  (2's comp)"  n_bits=48  bin_pt=0  quantization=Truncate  overflow=Wrap  latency=0  explicit_period=off  period=1  dbl_ovrd=off  show_param=off  inserted_by_tool=off  pipeline=off
      settings: xl_area=[0, 0, 0, 0, 0, 0, 0]
  Out1 : Outport
  wires:
  In1/1 -> ASlice/1, BSlice/1
  PrecB1/1 -> DSP48/2(b)
  PrecA1/1 -> DSP48/1(a)
  ASlice/1 -> PrecA1/1
  BSlice/1 -> PrecB1/1
  AlignP/1 -> UDType/1
  UDType/1 -> Out1/1
  ConvertP/1 -> AlignP/1
  In3/1 -> DSP48/3(opmode)
  In4/1 -> DSP48/4(subtract)
  In5/1 -> DSP48/5(carry_in)
  In6/1 -> DSP48/6(carry_in_sel)
  DSP48/1(P) -> ConvertP/1
  In2/1 -> Terminator/1
